simulink model "dos_attack"  (R2025b)
settings: Solver=ode4  StartTime=0.0  StopTime=50  FixedStep=dos_h  RelTol=1e-3
values from neighbouring files (symbols this model uses):
  dos_h = 0.01    [build_dos_attack.m]
  dos_seed = 2026    [build_dos_attack.m]
  dos_threshold = 0.2    [build_dos_attack.m]
settings Model: Creator=yuexi  LastModifiedBy=yuexi

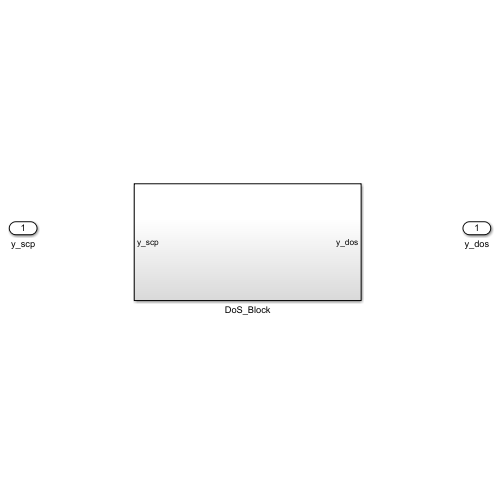
[thumbnail: Simulink's stored preview of the top-level diagram]
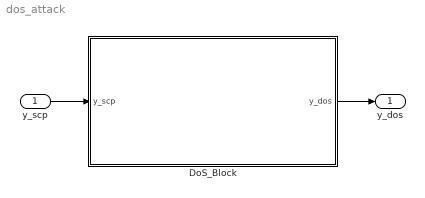
== system dos_attack ==
  y_scp : Inport
  DoS_Block : Subsystem
  y_dos : Outport
  wires:
  y_scp/1 -> DoS_Block/1(y_scp)
  DoS_Block/1(y_dos) -> y_dos/1

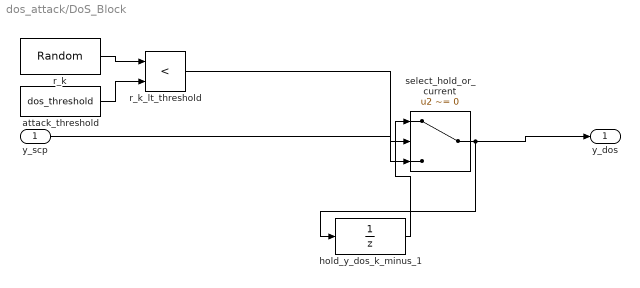
== system dos_attack/DoS_Block ==
  y_scp : Inport
  attack_threshold : Constant  Value=dos_threshold
  hold_y_dos_k_minus_1 : UnitDelay  SampleTime=dos_h  HasFrameUpgradeWarning=on
  r_k : UniformRandomNumber  Minimum=0  Seed=dos_seed  SampleTime=dos_h
  r_k_lt_threshold : RelationalOperator  Operator=<  OutDataTypeStr=boolean  RndMeth=Simplest  InputSameDT=off
  select_hold_or_current : Switch  Criteria=u2 ~= 0  Threshold=0.5  SaturateOnIntegerOverflow=off  InputSameDT=off
  y_dos : Outport
  wires:
  r_k/1 -> r_k_lt_threshold/1
  attack_threshold/1 -> r_k_lt_threshold/2
  hold_y_dos_k_minus_1/1 -> select_hold_or_current/1
  r_k_lt_threshold/1 -> select_hold_or_current/2
  y_scp/1 -> select_hold_or_current/3
  select_hold_or_current/1 -> y_dos/1, hold_y_dos_k_minus_1/1
